simulink model "ehvLogic"  (R2024a)
settings: Solver=FixedStepDiscrete  StartTime=0.0  StopTime=10.0  FixedStep=0.1  RelTol=1e-3  EnableMultiTasking=on
settings Model: Creator=farza  LastModifiedBy=farza
settings SolverCC: AlgebraicLoopSolver=TrustRegion  AutoInsertRateTranBlk=on
settings DataIOCC: LimitDataPoints=on
settings OptimizationCC: LifeSpan=inf
settings DebuggingCC: UnconnectedInputMsg=warning  UnconnectedOutputMsg=warning  UnconnectedLineMsg=warning  AllowSymbolicDim=off  SFUnexpectedBacktrackingDiag=warning  SFNoUnconditionalDefaultTransitionDiag=warning  SFExecutionAtInitializationDiag=none  ArithmeticOperatorsInVariantConditions=warning
settings ModelReferenceCC: EnableRefExpFcnMdlSchedulingChecks=on
settings SFSimCC: SimUseLocalCustomCode=off  CustomCodeUndefinedFunction=UseInterfaceOnly
settings RTWCC: RTWUseLocalCustomCode=off  GPUComputeCapability=3.5  DLArmComputeVersion=19.05
settings CodeAppCC: StateflowObjectComments=on
settings GRTTargetCC: TargetLangStandard=C89/C90 (ANSI)
settings ConfigComp: CovMetricSettings=dw  CovSaveCumulativeToWorkspaceVar=on  CovSaveSingleToWorkspaceVar=on  CovExternalEMLEnable=off  CovSFcnEnable=off

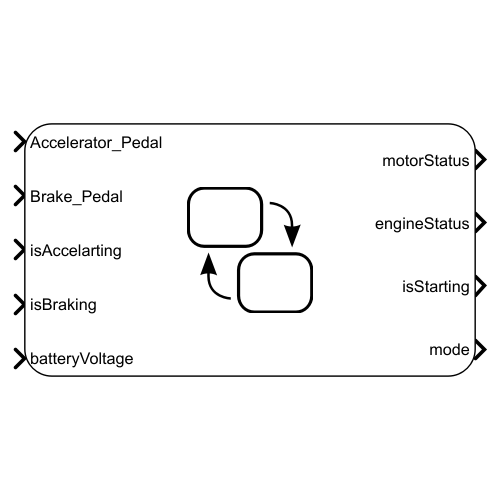
[thumbnail: Simulink's stored preview of the top-level diagram]
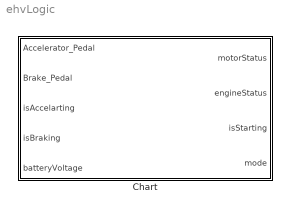
== system ehvLogic ==
  Chart : Stateflow chart  TreatAsAtomicUnit=on

== stateflow chart ehvLogic/Chart ==
  state Battery
    entry:
    enginStatus=0
    motorStatus=1
    mode=1
    batteryStatus=1
    during:
    batteryVoltage=batteryVoltage-SOC
    %battery provides starting
  state ICE
    entry:
    engineStatus=1
    motorStatus=1
    batteryStatus=0
    mode=2
    during:
  (default) -> Battery : Start
  Battery -> ICE : [Accelerator_Pedal>0.5 && Brake_Pedal<0.1]{engineStatus=1}
  data: Accelerator_Pedal input; Brake_Pedal input; isAccelarting input; isBraking input; motorStatus output; engineStatus output; isStarting output; batteryVoltage input; mode output
